simulink model "ANC_3"  (R2016b)
settings: Solver=VariableStepAuto  StartTime=0.0  StopTime=100.0  RelTol=1e-3
libraries: dspvision x1, audiosources x1, dspadpt3 x1, dspsrcs4 x1, dspobslib x1
settings Model: Creator=Ernest  LastModifiedBy=10458

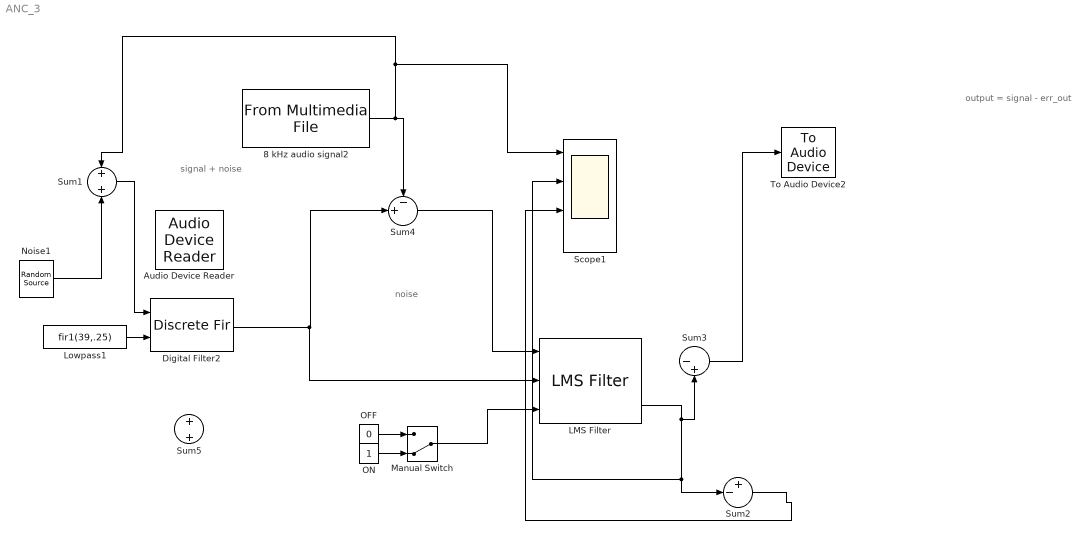
== system ANC_3 ==
  note: output = signal - err_out
  note: noise
  note: signal + noise
  8 kHz audio signal2 : dspvision/From Multimedia File  inputFilename=D:\Google Drive\Homework\Signals and Systems\Project\SingalChannelLiberation.wav  loop=on  numPlays=inf  outputStreams=Audio only  videoDataType=single  audioDataType=single  inheritSampleTime=on  userDefinedSampleTime=1/250  noAudioOutput=off  isIntensityVideo=off  fourcc=RGB  colorVideoFormat=Separate color signals  outputEOF=off  dataOrg=Column-major  audioFrameSize=1024  computeAudioFrameSize=off  outSamplingMode=Sample based
  Audio Device Reader : audiosources/Audio Device Reader  Driver=DirectSound  Device=Default  SampleRate=44100  NumChannels=1  SamplesPerFrame=128  BitDepth=16-bit integer  NumBuffers=10  DefaultInputChannelMapping=on  InputChannelMapping=1:2  OutputNumOverrunSamples=off  OutputDataType=double  DriverIdx=1  DeviceWarnFlag=''
  Digital Filter2 : DiscreteFir  CoefSource=Input port  Coefficients=[1 2]  InputProcessing=Columns as channels (frame based)  AccumDataTypeStr=Inherit: Same as product output  OutDataTypeStr=Inherit: Same as input
      settings: InputPortMap=u0,u1
  LMS Filter : dspadpt3/LMS Filter  Algo=LMS  L=32  stepflag=Dialog  mu=0.0008  leakage=1.0  ic=0  Adapt=on  resetflag=None  weights=off  secondCoeffMode=User-defined  secondCoeffWordLength=2  secondCoeffFracLength=15  accum2Mode=User-defined  accum2FracLength=20  prodOutput2Mode=User-defined  prodOutput2FracLength=20  prodOutput3Mode=User-defined  prodOutput3FracLength=20  prodOutput4Mode=User-defined  prodOutput4FracLength=20  quotientMode=User-defined  quotientFracLength=20  roundingMode=Floor  overflowMode=off  addnparflag=off
  Lowpass1 : Constant  Value=fir1(39,.25)  OutDataTypeStr=Inherit: Inherit via back propagation
  Manual Switch : ManualSwitch  CurrentSetting=0
  Noise1 : dspsrcs4/Random Source  SrcType=Gaussian  NormMethod=Sum of uniform values  CltLength=5  MinVal=-1  MaxVal=1  MeanVal=0  VarVal=10  RepMode=Not repeatable  rawSeed=[23341]  IsInherit=off  SampMode=Discrete  SampTime=1/44100  SampFrame=1024  DataType=Single  OutComplex=Real  OutputFrames=off
  OFF : Constant  Value=0
  ON : Constant
  Scope1 : Scope  NumInputPorts=4
  Sum1 : Sum  Inputs=+|+
  Sum2 : Sum  Inputs=+-|
  Sum3 : Sum  Inputs=|-+
  Sum4 : Sum  Inputs=-+|
  Sum5 : Sum  Inputs=+|+
  To Audio Device2 : dspobslib/To Audio Device  deviceName=Default  inheritSampleRate=on  sampleRate=44100  deviceDatatype=Determine from input data type  autoBufferSize=on  bufferSize=4096  queueDuration=1.0  defaultOutputChannelMapping=on  outputChannelMapping=1:2  outputNumUnderrunSamples=off
  wires:
  OFF/1 -> Manual Switch/1
  ON/1 -> Manual Switch/2
  Manual Switch/1 -> LMS Filter/3
  LMS Filter/2 -> Sum3/2, Scope1/2, Sum2/2
  Noise1/1 -> Sum1/2
  Sum4/1 -> LMS Filter/1
  Lowpass1/1 -> Digital Filter2/2
  Sum2/1 -> Scope1/3
  8 kHz audio signal2/1 -> Scope1/1, Sum1/1, Sum4/1
  Sum3/1 -> To Audio Device2/1
  Sum1/1 -> Digital Filter2/1
  Digital Filter2/1 -> LMS Filter/2, Sum4/2
